simulink model "obiekt_regulator"  (Simulink 7.4)
settings: Solver=ode45  StartTime=0.0  StopTime=100.0  RelTol=1e-3
values from neighbouring files (symbols this model uses):
  Kp = 0.95/abs(a)    [DobierzNastawy.m]
  L = [3]    [Symuluj.m]
  M = [2, 1, 1]    [Symuluj.m]
  SPS = 10    [Symuluj.m]
  step_ = 1e-2    (= 0.01)    [TestujObiekt.m]    (also in TestujRegulator.m)
  step_time = 10    [TestujRegulator.m]
  T = [0: 1/SPS : N/SPS - 1/SPS]    [GeneratorWeWy.m]    (also in Skok.m; Symuluj.m = 0.3)
  Td = 0.4*T0    [DobierzNastawy.m]
  Ti = 2.4*T0    [DobierzNastawy.m]
undefined symbols (not defined in the file or in its folder): DiscIntNeverNeededParam
libraries: dspsigops x1, simulink x1
settings Model: Creator=Konrad  LastModifiedBy=Konrad

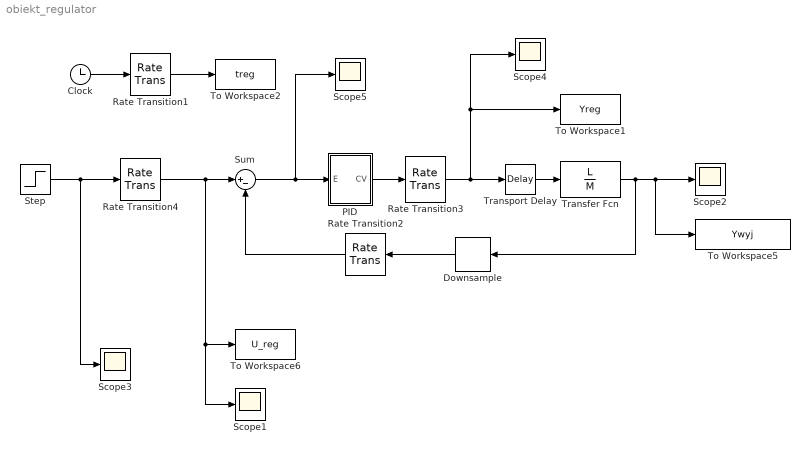
== system obiekt_regulator ==
  Clock : Clock
      settings: Decimation=10
  Downsample : dspsigops/Downsample  N=1/step_ / SPS  phase=0  ic=0  smode=Force single rate  fmode=Maintain input frame size
  PID : Subsystem  mask{Kp=Kp, Ti=Ti, Td=Td}
  Rate Transition1 : RateTransition  OutPortSampleTime=1/SPS
  Rate Transition2 : RateTransition  OutPortSampleTime=1/SPS
  Rate Transition3 : RateTransition
  Rate Transition4 : RateTransition  OutPortSampleTime=1/SPS
  Scope{1..5} (5 alike) : Scope
      Scope3 settings: SaveName=ScopeData2
      Scope4 settings: SaveName=ScopeData3
      Scope5 settings: SaveName=ScopeData4
  Step : Step  Time=step_time  SampleTime=1/SPS
  Sum : Sum  Inputs=|+-  OutDataType=fixdt(1, 16)  OutScaling=2^0
  To Workspace1 : ToWorkspace  VariableName=Yreg  SampleTime=-1  SaveFormat=Array
  To Workspace2 : ToWorkspace  VariableName=treg  SampleTime=1/SPS  SaveFormat=Array
  To Workspace5 : ToWorkspace  VariableName=Ywyj  SampleTime=-1  SaveFormat=Array
  To Workspace6 : ToWorkspace  VariableName=U_reg  SampleTime=-1  SaveFormat=Array
  Transfer Fcn : TransferFcn  Numerator=L  Denominator=M
  Transport Delay : TransportDelay  DelayTime=T
  wires:
  Clock/1 -> Rate Transition1/1
  Transfer Fcn/1 -> To Workspace5/1, Scope2/1, Downsample/1
  Transport Delay/1 -> Transfer Fcn/1
  Rate Transition1/1 -> To Workspace2/1
  Step/1 -> Scope3/1, Rate Transition4/1
  PID/1(CV) -> Rate Transition3/1
  Sum/1 -> PID/1(E), Scope5/1
  Rate Transition4/1 -> Scope1/1, To Workspace6/1, Sum/1
  Rate Transition3/1 -> Transport Delay/1, Scope4/1, To Workspace1/1
  Downsample/1 -> Rate Transition2/1
  Rate Transition2/1 -> Sum/2

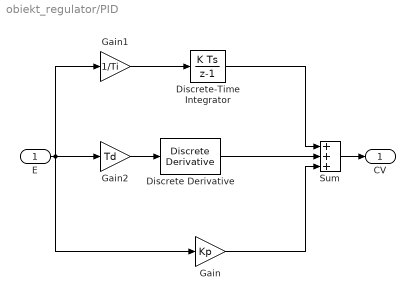
== system obiekt_regulator/PID ==
  E : Inport
  Discrete Derivative : simulink/Discrete/Discrete Derivative  SystemSampleTime=-1  gainval=1  ICPrevScaledInput=0.0  OutMin=[]  OutMax=[]  OutDataType=fixdt(1, 16)  OutScaling=2^-10  DoSatur=off
  Discrete-Time Integrator : DiscreteIntegrator  gainval=1  SampleTime=-1  OutDataType=fixdt(1, 16)  OutScaling=2^0  ICPrevOutput=DiscIntNeverNeededParam  ICPrevScaledInput=DiscIntNeverNeededParam
  Gain : Gain  Gain=Kp  ParameterDataType=fixdt(1, 16)  ParameterScaling=2^0  OutDataType=fixdt(1, 16)  OutScaling=2^0
  Gain1 : Gain  Gain=1/Ti  ParameterDataType=fixdt(1, 16)  ParameterScaling=2^0  OutDataType=fixdt(1, 16)  OutScaling=2^0
  Gain2 : Gain  Gain=Td  ParameterDataType=fixdt(1, 16)  ParameterScaling=2^0  OutDataType=fixdt(1, 16)  OutScaling=2^0
  Sum : Sum  Inputs=|+|+|+|  OutDataType=fixdt(1, 16)  OutScaling=2^0
  CV : Outport
  wires:
  E/1 -> Gain/1, Gain1/1, Gain2/1
  Discrete Derivative/1 -> Sum/2
  Gain/1 -> Sum/3
  Discrete-Time Integrator/1 -> Sum/1
  Sum/1 -> CV/1
  Gain1/1 -> Discrete-Time Integrator/1
  Gain2/1 -> Discrete Derivative/1
